simulink model "lab4"  (R2023a)
settings: Solver=VariableStepAuto  StartTime=0.0  StopTime=10.0  RelTol=1e-3
undefined symbols (not defined in the file): DiscIntNeverNeededParam
libraries: simulink x2
settings Model: Creator=Nitiz Khanal  LastModifiedBy=Nitiz Khanal

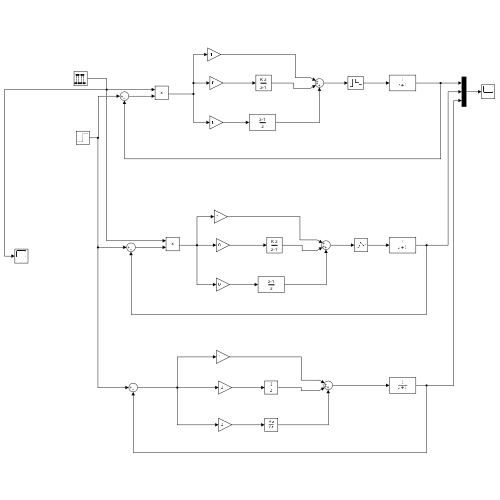
[thumbnail: Simulink's stored preview of the top-level diagram]
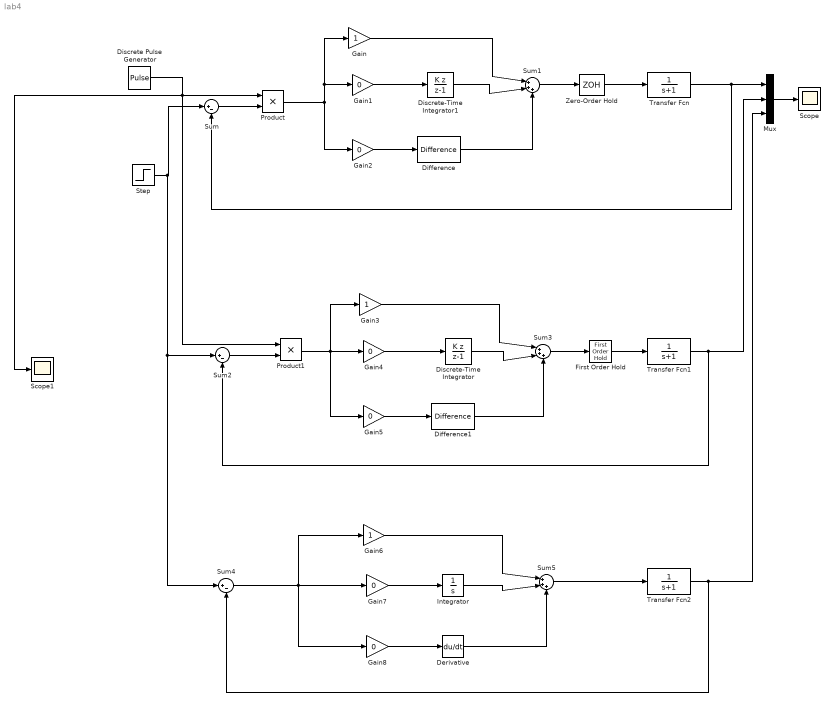
== system lab4 ==
  Derivative : Derivative
  Difference : simulink/Discrete/Difference  ICPrevInput=0.0  OutMin=[]  OutMax=[]  OutDataType=fixdt(1, 16)  OutScaling=2^-10  DoSatur=off
  Difference1 : simulink/Discrete/Difference  ICPrevInput=0.0  OutMin=[]  OutMax=[]  OutDataType=fixdt(1, 16)  OutScaling=2^-10  DoSatur=off
  Discrete Pulse Generator : DiscretePulseGenerator  Period=5  PulseWidth=5
  Discrete-Time Integrator : DiscreteIntegrator  IntegratorMethod=Accumulation: Backward Euler  SampleTime=-1  IgnoreLimit=on  ICPrevOutput=DiscIntNeverNeededParam  ICPrevScaledInput=DiscIntNeverNeededParam
  Discrete-Time Integrator1 : DiscreteIntegrator  IntegratorMethod=Accumulation: Backward Euler  SampleTime=-1  ICPrevOutput=DiscIntNeverNeededParam  ICPrevScaledInput=DiscIntNeverNeededParam
  First Order Hold : FirstOrderHold  ErrorTolerance=0  AllowContinuousInput=on
  Gain : Gain
  Gain{1..2,4..5,7..8} (6 alike) : Gain  Gain=0
  Gain3 : Gain
  Gain6 : Gain
  Integrator : Integrator
  Mux : Mux  Inputs=3
  Product : Product
  Product1 : Product
  Scope : Scope
  Scope1 : Scope
  Step : Step  SampleTime=0.5
  Sum : Sum  Inputs=|+-
  Sum1 : Sum  Inputs=|+++
  Sum2 : Sum  Inputs=|+-
  Sum3 : Sum  Inputs=|+++
  Sum4 : Sum  Inputs=|+-
  Sum5 : Sum  Inputs=|+++
  Transfer Fcn : TransferFcn  Denominator=[1 1]
  Transfer Fcn1 : TransferFcn  Denominator=[1 1]
  Transfer Fcn2 : TransferFcn  Denominator=[1 1]
  Zero-Order Hold : ZeroOrderHold  SampleTime=-1
  wires:
  Step/1 -> Sum4/1, Sum2/1, Sum/1
  Sum/1 -> Product/2
  Product/1 -> Gain/1, Gain1/1, Gain2/1
  Gain/1 -> Sum1/1
  Gain1/1 -> Discrete-Time Integrator1/1
  Discrete-Time Integrator1/1 -> Sum1/2
  Sum1/1 -> Zero-Order Hold/1
  Zero-Order Hold/1 -> Transfer Fcn/1
  Transfer Fcn/1 -> Mux/1, Sum/2
  Sum2/1 -> Product1/2
  Product1/1 -> Gain3/1, Gain5/1, Gain4/1
  Gain3/1 -> Sum3/1
  Gain4/1 -> Discrete-Time Integrator/1
  Gain5/1 -> Difference1/1
  Difference1/1 -> Sum3/3
  First Order Hold/1 -> Transfer Fcn1/1
  Mux/1 -> Scope/1
  Transfer Fcn1/1 -> Mux/2, Sum2/2
  Transfer Fcn2/1 -> Mux/3, Sum4/2
  Sum5/1 -> Transfer Fcn2/1
  Sum4/1 -> Gain8/1, Gain7/1, Gain6/1
  Gain7/1 -> Integrator/1
  Gain8/1 -> Derivative/1
  Gain6/1 -> Sum5/1
  Integrator/1 -> Sum5/2
  Derivative/1 -> Sum5/3
  Sum3/1 -> First Order Hold/1
  Difference/1 -> Sum1/3
  Gain2/1 -> Difference/1
  Discrete-Time Integrator/1 -> Sum3/2
  Discrete Pulse Generator/1 -> Scope1/1, Product1/1, Product/1
